simulink model "Car_model"  (Simulink 8.2)
settings: Solver=ode45  StartTime=0.0  StopTime=10.0  RelTol=1e-3
values from neighbouring files (symbols this model uses):
  a = 1.06    [voertuigdata.m]
  b = L-a    (= 1.6)    [voertuigdata.m]
  Cy_achter = B2*C2*D2    [voertuigdata.m]
  Cy_voor = B1*C1*D1    [voertuigdata.m]
  g = 9.81    [voertuigdata.m]
  J = 1850    [voertuigdata.m]
  m = 1150    [voertuigdata.m]
  v = v/3.6    (= 22.2222222222)    [voertuigdata.m]
settings Model: Creator=879618  LastModifiedBy=275666
settings DataIOCC: SignalLoggingSaveFormat=Dataset
settings DebuggingCC: FcnCallInpInsideContextMsg=EnableAllAsError
settings GRTTargetCC: CombineOutputUpdateFcns=on  GRTInterface=off

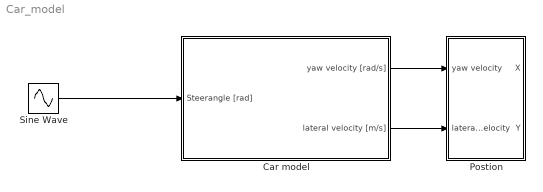
== system Car_model ==
  Car model : Subsystem
  Postion : Subsystem
  Sine Wave : Sin  Amplitude=0.2  SampleTime=0
  wires:
  Car model/1(yaw velocity [rad/s]) -> Postion/1(yaw velocity)
  Car model/2(lateral velocity [m/s]) -> Postion/2(lateral velocity)
  Sine Wave/1 -> Car model/1(Steerangle [rad])

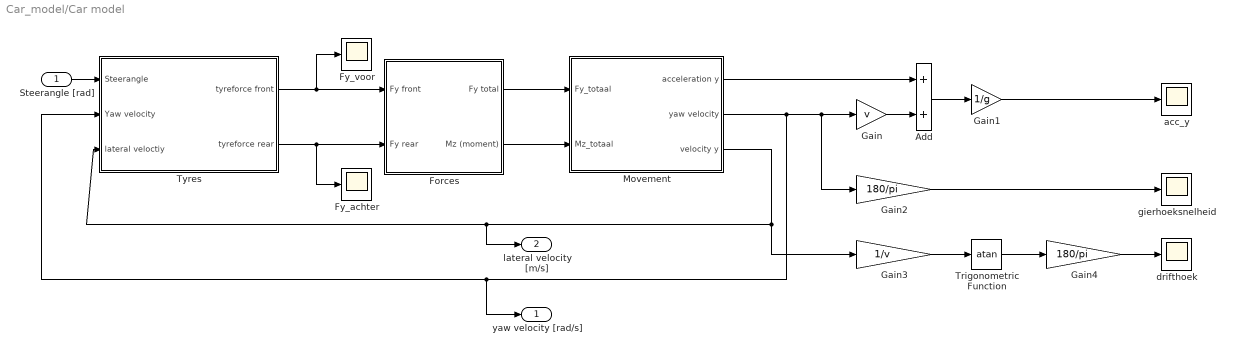
== system Car_model/Car model ==
  Steerangle [rad] : Inport
  Add : Sum
  Forces : Subsystem
  Fy_achter : Scope
      settings: SaveName=Fy_achter
  Fy_voor : Scope
      settings: TimeRange=10  SaveName=Fy_voor
  Gain : Gain  Gain=v
  Gain1 : Gain  Gain=1/g
  Gain2 : Gain  Gain=180/pi
  Gain3 : Gain  Gain=1/v
  Gain4 : Gain  Gain=180/pi
  Movement : Subsystem
  Trigonometric Function : Trigonometry  Operator=atan
  Tyres : Subsystem
  acc_y : Scope
      settings: TimeRange=10  YMin=-1  YMax=1  SaveName=acc_y
  drifthoek : Scope
      settings: SaveName=beta
  gierhoeksnelheid : Scope
      settings: SaveName=yaw_rate
  yaw velocity [rad/s] : Outport
  lateral velocity [m/s] : Outport  Port=2
  wires:
  Tyres/1(tyreforce front) -> Fy_voor/1, Forces/1(Fy front)
  Tyres/2(tyreforce rear) -> Fy_achter/1, Forces/2(Fy rear)
  Forces/2(Mz (moment)) -> Movement/2(Mz_totaal)
  Forces/1(Fy total) -> Movement/1(Fy_totaal)
  Movement/1(acceleration y) -> Add/1
  Gain/1 -> Add/2
  Add/1 -> Gain1/1
  Gain3/1 -> Trigonometric Function/1
  Trigonometric Function/1 -> Gain4/1
  Gain1/1 -> acc_y/1
  Gain4/1 -> drifthoek/1
  Movement/2(yaw velocity) -> Gain/1, Gain2/1, yaw velocity [rad/s]/1, Tyres/2(Yaw velocity)
  Movement/3(velocity y) -> Gain3/1, Tyres/3(lateral veloctiy), lateral velocity [m/s]/1
  Steerangle [rad]/1 -> Tyres/1(Steerangle)
  Gain2/1 -> gierhoeksnelheid/1

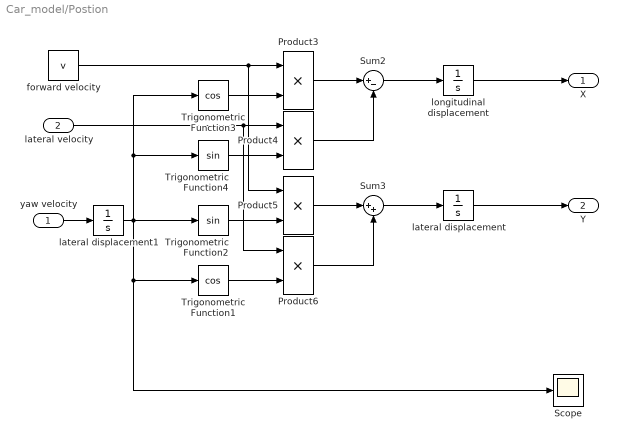
== system Car_model/Postion ==
  yaw velocity : Inport
  lateral velocity : Inport  Port=2
  Product{3..6} (4 alike) : Product  RndMeth=Zero
  Scope : Scope
  Sum2 : Sum  Inputs=|+-
  Sum3 : Sum  Inputs=|++
  Trigonometric Function1 : Trigonometry  Operator=cos
  Trigonometric Function2 : Trigonometry
  Trigonometric Function3 : Trigonometry  Operator=cos
  Trigonometric Function4 : Trigonometry
  forward velocity : Constant  Value=v
  lateral displacement : Integrator
  lateral displacement1 : Integrator
  longitudinal displacement : Integrator
  X : Outport
  Y : Outport  Port=2
  wires:
  longitudinal displacement/1 -> X/1
  lateral displacement/1 -> Y/1
  yaw velocity/1 -> lateral displacement1/1
  forward velocity/1 -> Product3/1, Product5/1
  lateral velocity/1 -> Product4/1, Product6/1
  Trigonometric Function4/1 -> Product4/2
  Trigonometric Function3/1 -> Product3/2
  Trigonometric Function2/1 -> Product5/2
  Trigonometric Function1/1 -> Product6/2
  Sum3/1 -> lateral displacement/1
  Product6/1 -> Sum3/2
  Product5/1 -> Sum3/1
  Sum2/1 -> longitudinal displacement/1
  Product4/1 -> Sum2/2
  Product3/1 -> Sum2/1
  lateral displacement1/1 -> Trigonometric Function2/1, Trigonometric Function4/1, Trigonometric Function3/1, Trigonometric Function1/1, Scope/1

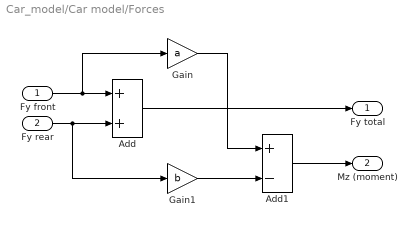
== system Car_model/Car model/Forces ==
  Fy front : Inport
  Fy rear : Inport  Port=2
  Add : Sum
  Add1 : Sum  Inputs=+-
  Gain : Gain  Gain=a
  Gain1 : Gain  Gain=b
  Fy total : Outport
  Mz (moment) : Outport  Port=2
  wires:
  Fy front/1 -> Gain/1, Add/1
  Fy rear/1 -> Gain1/1, Add/2
  Gain/1 -> Add1/1
  Gain1/1 -> Add1/2
  Add/1 -> Fy total/1
  Add1/1 -> Mz (moment)/1

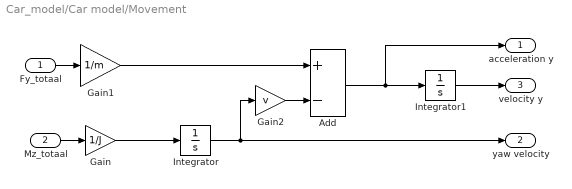
== system Car_model/Car model/Movement ==
  Fy_totaal : Inport
  Mz_totaal : Inport  Port=2
  Add : Sum  Inputs=+-
  Gain : Gain  Gain=1/J
  Gain1 : Gain  Gain=1/m
  Gain2 : Gain  Gain=v
  Integrator : Integrator
  Integrator1 : Integrator
  acceleration y : Outport
  yaw velocity : Outport  Port=2
  velocity y : Outport  Port=3
  wires:
  Gain/1 -> Integrator/1
  Gain1/1 -> Add/1
  Integrator/1 -> Gain2/1, yaw velocity/1
  Gain2/1 -> Add/2
  Add/1 -> acceleration y/1, Integrator1/1
  Fy_totaal/1 -> Gain1/1
  Integrator1/1 -> velocity y/1
  Mz_totaal/1 -> Gain/1

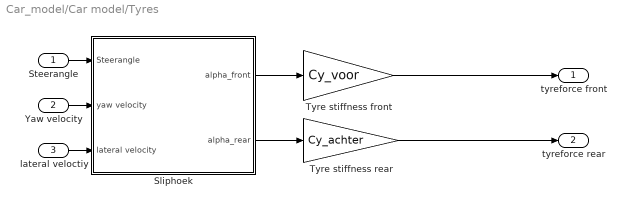
== system Car_model/Car model/Tyres ==
  Steerangle : Inport
  Yaw velocity : Inport  Port=2
  lateral veloctiy : Inport  Port=3
  Sliphoek : Subsystem
  Tyre stiffness front : Gain  Gain=Cy_voor
  Tyre stiffness rear : Gain  Gain=Cy_achter
  tyreforce front : Outport
  tyreforce rear : Outport  Port=2
  wires:
  Sliphoek/2(alpha_rear) -> Tyre stiffness rear/1
  Sliphoek/1(alpha_front) -> Tyre stiffness front/1
  Steerangle/1 -> Sliphoek/1(Steerangle)
  Yaw velocity/1 -> Sliphoek/2(yaw velocity)
  lateral veloctiy/1 -> Sliphoek/3(lateral velocity)
  Tyre stiffness front/1 -> tyreforce front/1
  Tyre stiffness rear/1 -> tyreforce rear/1

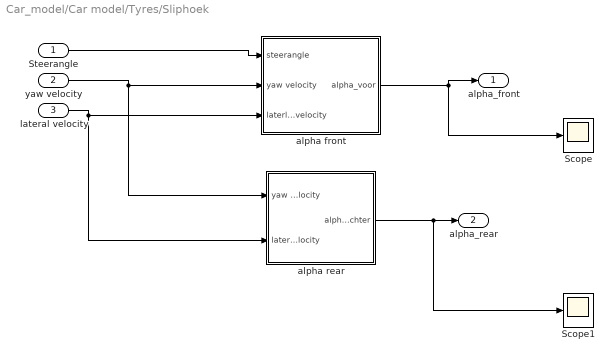
== system Car_model/Car model/Tyres/Sliphoek ==
  Steerangle : Inport
  yaw velocity : Inport  Port=2
  lateral velocity : Inport  Port=3
  Scope : Scope
      settings: TimeRange=10  YMin=-0.004  YMax=0  SaveName=alpha_voor
  Scope1 : Scope
      settings: TimeRange=10  YMin=-0.004  YMax=0  SaveName=alpha_achter
  alpha front : Subsystem
  alpha rear : Subsystem
  alpha_front : Outport
  alpha_rear : Outport  Port=2
  wires:
  yaw velocity/1 -> alpha front/2(yaw velocity), alpha rear/1(yaw velocity)
  lateral velocity/1 -> alpha front/3(laterlal velocity), alpha rear/2(lateral velocity)
  Steerangle/1 -> alpha front/1(steerangle)
  alpha front/1(alpha_voor) -> alpha_front/1, Scope/1
  alpha rear/1(alpha_achter) -> alpha_rear/1, Scope1/1

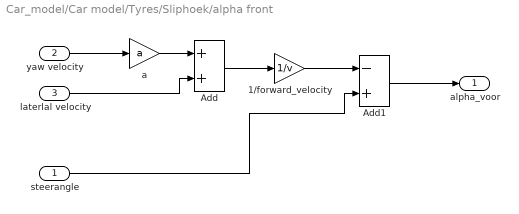
== system Car_model/Car model/Tyres/Sliphoek/alpha front ==
  steerangle : Inport
  yaw velocity : Inport  Port=2
  laterlal velocity : Inport  Port=3
  1/forward_velocity : Gain  Gain=1/v
  Add : Sum
  Add1 : Sum  Inputs=-+
  a : Gain  Gain=a
  alpha_voor : Outport
  wires:
  a/1 -> Add/1
  Add/1 -> 1/forward_velocity/1
  yaw velocity/1 -> a/1
  laterlal velocity/1 -> Add/2
  steerangle/1 -> Add1/2
  Add1/1 -> alpha_voor/1
  1/forward_velocity/1 -> Add1/1

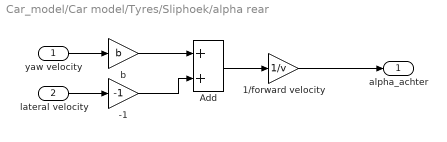
== system Car_model/Car model/Tyres/Sliphoek/alpha rear ==
  yaw velocity : Inport
  lateral velocity : Inport  Port=2
  -1 : Gain  Gain=-1
  1/forward velocity : Gain  Gain=1/v
  Add : Sum
  b : Gain  Gain=b
  alpha_achter : Outport
  wires:
  lateral velocity/1 -> -1/1
  yaw velocity/1 -> b/1
  1/forward velocity/1 -> alpha_achter/1
  Add/1 -> 1/forward velocity/1
  b/1 -> Add/1
  -1/1 -> Add/2
